simulink model "autonomous_takeoff_landing"  (Simulink 7.8)
settings: Solver=ode3  StartTime=0.0  StopTime=10.0  FixedStep=0.01  RelTol=1e-3
values from neighbouring files (symbols this model uses):
  Bkrit = 1    [parameter_ZA.m]
  Bsafe = 3    [parameter_ZA.m]
  Bstart = 5    [parameter_ZA.m]
  C_wxy = 1/2*A_xy*rho*c_w    (= 0.01986730725)    [parameter_QK.m]
  C_wz = 1/2*A_z*rho*c_w    (= 0.141396406537)    [parameter_QK.m]
  CT0 = 0.0133    [parameter_QK.m]
  CT1 = -0.0100    (= -0.01)    [parameter_QK.m]
  CT2 = 0.0081    [parameter_QK.m]
  CT3 = -0.0350    (= -0.035)    [parameter_QK.m]
  dhSinkflug = .05    (= 0.05)    [parameter_ZA.m]
  dhZulSinkflug = .05    (= 0.05)    [parameter_ZA.m]
  dSchubLanden = .05    (= 0.05)    [parameter_ZA.m]
  dSchubStart = .01    (= 0.01)    [parameter_ZA.m]
  dt = 0.01    [init.m]
  dtStart = .2    (= 0.2)    [parameter_ZA.m]
  g = 9.81    [parameter_QK.m]    (also in zulwin.m = sin(beta+pi/4)*LGB/2)
  hFlug = 1    [parameter_ZA.m]
  hLanden = LGH*4    (= 0.6)    [parameter_ZA.m]
  l_m = 0.2775    [parameter_QK.m]    (also in zulwin.m)
  LGH = 0.15    [init.m]    (also in parameter_ZA.m)
  m = 1.316    [parameter_QK.m]
  R = 0.1269    [parameter_QK.m]    (also in zulwin.m)
  rho = 1.225    [parameter_QK.m]
  SchubRun = .2    (= 0.2)    [parameter_ZA.m]
  SchubStart = 0.65    [parameter_ZA.m]
  tAnlauf = 2.5    [parameter_ZA.m]
  twc = .1    (= 0.1)    [parameter_ZA.m]
  z_m = -0.02    [parameter_QK.m]
  zpLanden = .05    (= 0.05)    [parameter_ZA.m]
  zpStart = .1    (= 0.1)    [parameter_ZA.m]
  zul_dmotor = 25    [parameter_ZA.m]
  zul_dp = .15    (= 0.15)    [parameter_ZA.m]
  zul_dwmax = 0.8    [parameter_ZA.m]
  zul_w = 2.5    [parameter_ZA.m]
  zul_win = .15    (= 0.15)    [parameter_ZA.m]
undefined symbols (not defined in the file or in its folder): Newton, Raphson
libraries: simulink x28, orocos_taskcontext x18, powerlib_extras x6, aerolibutil x4, aerolibtransform2 x1, dspmtrx3 x1
settings Model: Creator=roedelsperger  LastModifiedBy=uav
settings DebuggingCC: FcnCallInpInsideContextMsg=Use local settings
settings RTWCC: SystemTargetFile=orocos.tlc  TemplateMakefile=orocos.tmf  Description=Linux Orocos Target  ProcessScript=orocos_make_rtw_hook
settings STFCustomTargetCC: ModelReferenceCompliant=off  MatFileLogging=on  SystemTargetFile=orocos.tlc

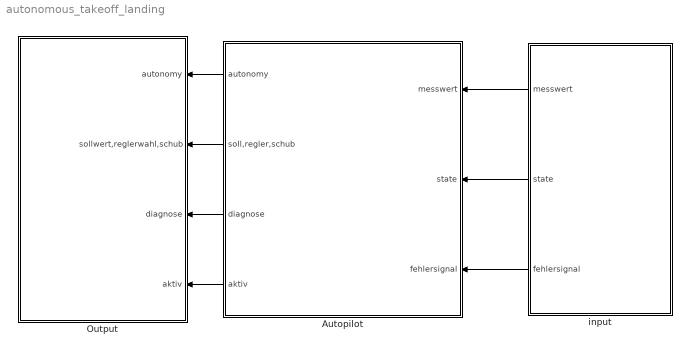
== system autonomous_takeoff_landing ==
  Autopilot : Subsystem
  Output : Subsystem
  input : Subsystem
  wires:
  input/1(messwert) -> Autopilot/1(messwert)
  input/2(state) -> Autopilot/2(state)
  Autopilot/1(autonomy) -> Output/1(autonomy)
  Autopilot/2(soll,regler,schub) -> Output/2(sollwert,reglerwahl,schub)
  Autopilot/3(diagnose) -> Output/3(diagnose)
  Autopilot/4(aktiv) -> Output/4(aktiv)
  input/3(fehlersignal) -> Autopilot/3(fehlersignal)

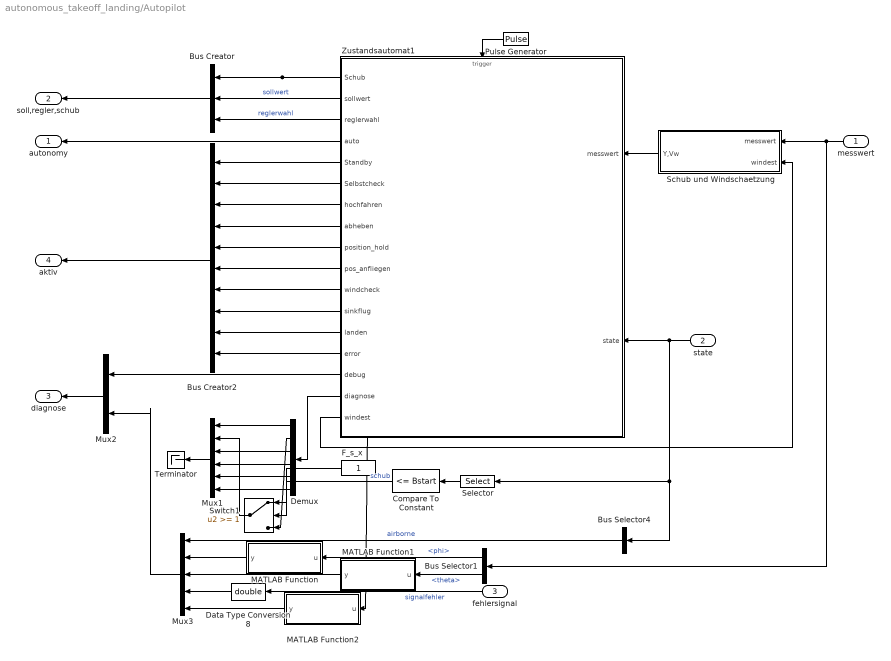
== system autonomous_takeoff_landing/Autopilot ==
  messwert : Inport
  state : Inport  Port=2
  fehlersignal : Inport  Port=3
  Bus Creator : BusCreator  Inputs=3
  Bus Creator2 : BusCreator  Inputs=10
  Bus Selector1 : BusSelector  OutputSignals=ptp.phi,ptp.theta
  Bus Selector4 : BusSelector  OutputSignals=signal5  OutputAsBus=on
  Compare To Constant : simulink/Logic and Bit Operations/Compare To Constant  relop=<=  const=Bstart  OutDataTypeStr=uint8
  Data Type Conversion8 : DataTypeConversion  OutDataTypeStr=double  RndMeth=Ceiling
  Demux : Demux  Outputs=6
  F_s_x : Constant
  MATLAB Function : MATLAB Function  TreatAsAtomicUnit=on
  MATLAB Function1 : MATLAB Function  TreatAsAtomicUnit=on
  MATLAB Function2 : MATLAB Function  TreatAsAtomicUnit=on
  Mux1 : Mux  Inputs=6
  Mux2 : Mux  Inputs=2
  Mux3 : Mux  Inputs=5
  Pulse Generator : DiscretePulseGenerator  PulseType=Time based  Period=0.02  PulseWidth=50
  Schub und Windschaetzung : Subsystem
  Selector : Selector  InputPortWidth=6  IndexOptions=Index vector (dialog)  Indices=[6]  OutputSizes=1
  Switch1 : Switch  Threshold=1
  Terminator : Terminator
  Zustandsautomat1 : Stateflow chart  TreatAsAtomicUnit=on
  autonomy : Outport
  soll,regler,schub : Outport  Port=2
  diagnose : Outport  Port=3
  aktiv : Outport  Port=4
  wires:
  messwert/1 -> Schub und Windschaetzung/1(messwert), Bus Selector1/1
  Pulse Generator/1 -> Zustandsautomat1/Trigger
  state/1 -> Zustandsautomat1/2(state), Selector/1, Bus Selector4/1
  Zustandsautomat1/1(Schub) -> Bus Creator/1, MATLAB Function2/1(u)  "schub"
  Zustandsautomat1/17(windest) -> Schub und Windschaetzung/2(windest)
  Demux/1 -> Mux1/1
  Demux/2 -> Switch1/3
  Switch1/1 -> Mux1/2
  Zustandsautomat1/16(diagnose) -> Demux/1
  Compare To Constant/1 -> Switch1/2
  Bus Creator/1 -> soll,regler,schub/1
  Zustandsautomat1/2(sollwert) -> Bus Creator/2  "sollwert"
  Zustandsautomat1/3(reglerwahl) -> Bus Creator/3  "reglerwahl"
  Zustandsautomat1/4(auto) -> autonomy/1
  Schub und Windschaetzung/1(Y,Vw) -> Zustandsautomat1/1(messwert)
  F_s_x/1 -> Switch1/1
  Selector/1 -> Compare To Constant/1
  Zustandsautomat1/5(Standby) -> Bus Creator2/1
  Zustandsautomat1/6(Selbstcheck) -> Bus Creator2/2
  Zustandsautomat1/7(hochfahren) -> Bus Creator2/3
  Zustandsautomat1/8(abheben) -> Bus Creator2/4
  Zustandsautomat1/9(position_hold) -> Bus Creator2/5
  Zustandsautomat1/10(pos_anfliegen) -> Bus Creator2/6
  Zustandsautomat1/11(windcheck) -> Bus Creator2/7
  Zustandsautomat1/12(sinkflug) -> Bus Creator2/8
  Zustandsautomat1/13(landen) -> Bus Creator2/9
  Zustandsautomat1/14(error) -> Bus Creator2/10
  Bus Creator2/1 -> aktiv/1
  Demux/3 -> Mux1/3
  Demux/4 -> Mux1/4
  Demux/5 -> Mux1/5
  Demux/6 -> Mux1/6
  Zustandsautomat1/15(debug) -> Mux2/1
  Mux2/1 -> diagnose/1
  Mux3/1 -> Mux2/2
  Mux1/1 -> Terminator/1
  fehlersignal/1 -> Data Type Conversion8/1  "signalfehler"
  Bus Selector4/1 -> Mux3/1  "airborne"
  Data Type Conversion8/1 -> Mux3/4
  MATLAB Function/1(y) -> Mux3/2
  Bus Selector1/1 -> MATLAB Function/1(u)  "<phi>"
  Bus Selector1/2 -> MATLAB Function1/1(u)  "<theta>"
  MATLAB Function1/1(y) -> Mux3/3
  MATLAB Function2/1(y) -> Mux3/5

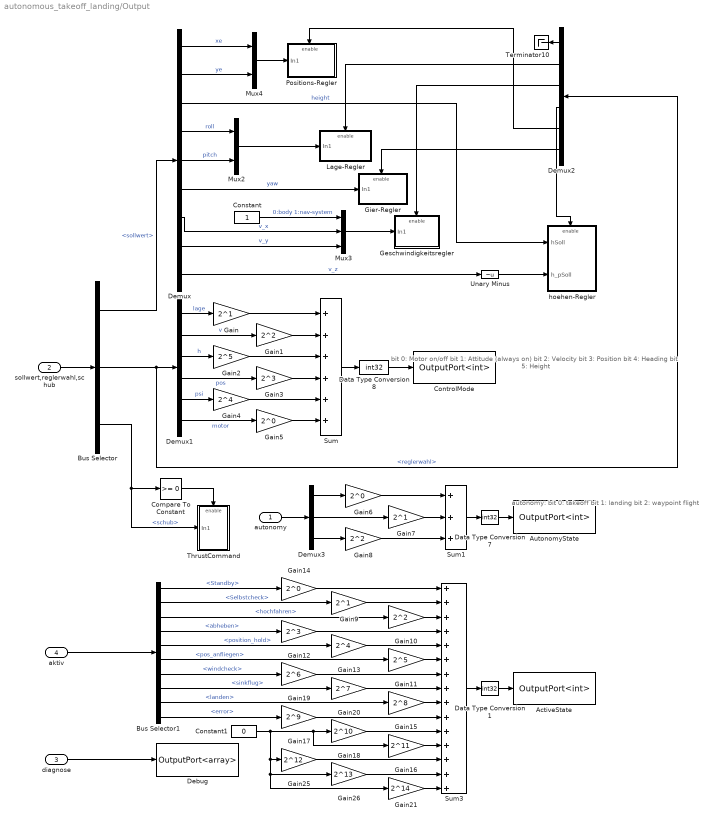
== system autonomous_takeoff_landing/Output ==
  note: bit 0: Motor on/off
      | bit 1: Attitude (always on)
      | bit 2: Velocity
      | bit 3: Position
      | bit 4: Heading
      | bit 5: Height
  note: autonomy:
      |   bit 0: takeoff
      |   bit 1: landing
      |   bit 2: waypoint flight
  autonomy : Inport
  sollwert,reglerwahl,schub : Inport  Port=2
  diagnose : Inport  Port=3
  aktiv : Inport  Port=4
  ActiveState : orocos_taskcontext/OutputPort<int>  dpdesc=Port's Description  dpvalue=0
      settings: AttributesFormatString=Value=%<dpvalue>
  AutonomyState : orocos_taskcontext/OutputPort<int>  dpdesc=Port's Description  dpvalue=0
      settings: AttributesFormatString=Value=%<dpvalue>
  Bus Selector : BusSelector  OutputSignals=sollwert,reglerwahl,schub
  Bus Selector1 : BusSelector  OutputSignals=Standby,Selbstcheck,hochfahren,abheben,position_hold,pos_anfliegen,windcheck,sinkflug,landen,error
  Compare To Constant : simulink/Logic and Bit Operations/Compare To Constant  relop=>=  const=0  OutDataTypeStr=uint8
  Constant : Constant
  Constant1 : Constant  Value=0
  ControlMode : orocos_taskcontext/OutputPort<int>  dpdesc=Port's Description  dpvalue=0
      settings: AttributesFormatString=Value=%<dpvalue>
  Data Type Conversion1 : DataTypeConversion  OutDataTypeStr=int32  RndMeth=Ceiling
  Data Type Conversion7 : DataTypeConversion  OutDataTypeStr=int32  RndMeth=Ceiling
  Data Type Conversion8 : DataTypeConversion  OutDataTypeStr=int32  RndMeth=Ceiling
  Debug : orocos_taskcontext/OutputPort<array>  dpdesc=Port's Description  dpvalue=[0.0]
      settings: AttributesFormatString=Value=%<dpvalue>
  Demux : Demux  Outputs=9
  Demux1 : Demux  Outputs=6
  Demux2 : Demux  Outputs=6
  Demux3 : Demux  Outputs=3
  Gain : Gain  Gain=2^1
  Gain1 : Gain  Gain=2^2
  Gain10 : Gain  Gain=2^2
  Gain11 : Gain  Gain=2^5
  Gain12 : Gain  Gain=2^3
  Gain13 : Gain  Gain=2^4
  Gain14 : Gain  Gain=2^0
  Gain15 : Gain  Gain=2^8
  Gain16 : Gain  Gain=2^11
  Gain17 : Gain  Gain=2^9
  Gain18 : Gain  Gain=2^10
  Gain19 : Gain  Gain=2^6
  Gain2 : Gain  Gain=2^5
  Gain20 : Gain  Gain=2^7
  Gain21 : Gain  Gain=2^14
  Gain25 : Gain  Gain=2^12
  Gain26 : Gain  Gain=2^13
  Gain3 : Gain  Gain=2^3
  Gain4 : Gain  Gain=2^4
  Gain5 : Gain  Gain=2^0
  Gain6 : Gain  Gain=2^0
  Gain7 : Gain  Gain=2^1
  Gain8 : Gain  Gain=2^2
  Gain9 : Gain  Gain=2^1
  Geschwindigkeitsregler : Subsystem
  Gier-Regler : Subsystem
  Lage-Regler : Subsystem
  Mux2 : Mux  Inputs=2
  Mux3 : Mux  Inputs=3
  Mux4 : Mux  Inputs=2
  Positions-Regler : Subsystem
  Sum : Sum  Inputs=++++++
  Sum1 : Sum  Inputs=+++
  Sum3 : Sum  Inputs=+++++++++++++++
  Terminator10 : Terminator
  ThrustCommand : Subsystem
  Unary Minus : UnaryMinus
  hoehen-Regler : Subsystem
  wires:
  sollwert,reglerwahl,schub/1 -> Bus Selector/1
  Bus Selector/1 -> Demux/1  "<sollwert>"
  Mux2/1 -> Lage-Regler/1(In1)
  Demux/4 -> Mux2/1  "roll"
  Demux/5 -> Mux2/2  "pitch"
  Demux/6 -> Gier-Regler/1(In1)  "yaw"
  Mux3/1 -> Geschwindigkeitsregler/1(In1)
  Constant/1 -> Mux3/1  "0:body 1:nav-system"
  Demux/7 -> Mux3/2  "v_x"
  Demux/8 -> Mux3/3  "v_y"
  Demux/3 -> hoehen-Regler/1(hSoll)  "height"
  Demux/9 -> Unary Minus/1  "v_z"
  Demux/1 -> Mux4/1  "xe"
  Demux/2 -> Mux4/2  "ye"
  Mux4/1 -> Positions-Regler/1(In1)
  Demux2/1 -> Terminator10/1
  Demux2/2 -> Lage-Regler/Enable
  Demux2/3 -> Geschwindigkeitsregler/Enable
  Demux2/4 -> hoehen-Regler/Enable
  Demux2/5 -> Positions-Regler/Enable
  Demux2/6 -> Gier-Regler/Enable
  Compare To Constant/1 -> ThrustCommand/Enable
  Bus Selector/2 -> Demux1/1, Demux2/1  "<reglerwahl>"
  Unary Minus/1 -> hoehen-Regler/2(h_pSoll)
  Demux1/1 -> Gain/1  "lage"
  Demux1/2 -> Gain1/1  "v"
  Demux1/3 -> Gain2/1  "h"
  Demux1/4 -> Gain3/1  "pos"
  Demux1/5 -> Gain4/1  "psi"
  Demux1/6 -> Gain5/1  "motor"
  Gain6/1 -> Sum1/1
  Gain7/1 -> Sum1/2
  Gain8/1 -> Sum1/3
  Sum1/1 -> Data Type Conversion7/1
  Demux3/1 -> Gain6/1
  Demux3/2 -> Gain7/1
  Demux3/3 -> Gain8/1
  autonomy/1 -> Demux3/1
  Bus Selector/3 -> Compare To Constant/1, ThrustCommand/1(In1)  "<schub>"
  Sum/1 -> Data Type Conversion8/1
  Data Type Conversion7/1 -> AutonomyState/1
  Data Type Conversion8/1 -> ControlMode/1
  Gain/1 -> Sum/1
  Gain1/1 -> Sum/2
  Gain2/1 -> Sum/3
  Gain3/1 -> Sum/4
  Gain4/1 -> Sum/5
  Gain5/1 -> Sum/6
  aktiv/1 -> Bus Selector1/1
  Sum3/1 -> Data Type Conversion1/1
  Data Type Conversion1/1 -> ActiveState/1
  Bus Selector1/1 -> Gain14/1  "<Standby>"
  Bus Selector1/2 -> Gain9/1  "<Selbstcheck>"
  Bus Selector1/3 -> Gain10/1  "<hochfahren>"
  Bus Selector1/4 -> Gain12/1  "<abheben>"
  Bus Selector1/5 -> Gain13/1  "<position_hold>"
  Bus Selector1/6 -> Gain11/1  "<pos_anfliegen>"
  Bus Selector1/7 -> Gain19/1  "<windcheck>"
  Bus Selector1/8 -> Gain20/1  "<sinkflug>"
  Bus Selector1/9 -> Gain15/1  "<landen>"
  Bus Selector1/10 -> Gain17/1  "<error>"
  Gain14/1 -> Sum3/1
  Gain9/1 -> Sum3/2
  Gain10/1 -> Sum3/3
  Gain12/1 -> Sum3/4
  Gain13/1 -> Sum3/5
  Gain11/1 -> Sum3/6
  Gain19/1 -> Sum3/7
  Gain20/1 -> Sum3/8
  Gain15/1 -> Sum3/9
  Gain17/1 -> Sum3/10
  Gain18/1 -> Sum3/11
  Gain16/1 -> Sum3/12
  Gain25/1 -> Sum3/13
  Gain26/1 -> Sum3/14
  Gain21/1 -> Sum3/15
  diagnose/1 -> Debug/1
  Constant1/1 -> Gain18/1, Gain16/1, Gain25/1, Gain26/1, Gain21/1

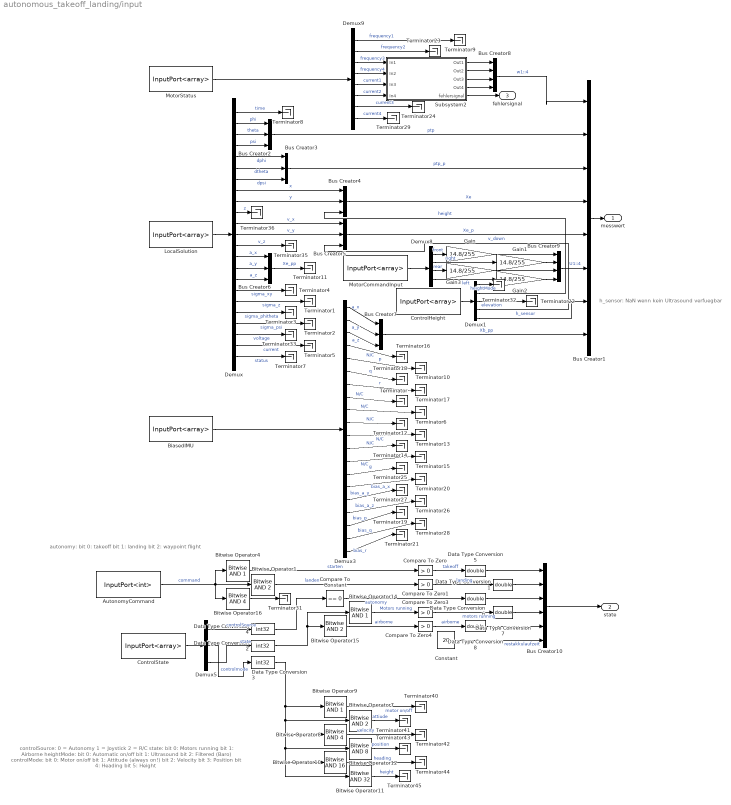
== system autonomous_takeoff_landing/input ==
  note: autonomy:
      |   bit 0: takeoff
      |   bit 1: landing
      |   bit 2: waypoint flight
  note: controlSource:
      |   0 = Autonomy
      |   1 = Joystick
      |   2 = R/C
      | state:
      |   bit 0: Motors running
      |   bit 1: Airborne
      | heightMode:
      |   bit 0: Automatic on/off
      |   bit 1: Ultrasound
      |   bit 2: Filtered (Baro)
      | controlMode:
      |   bit 0: Motor on/off
      |   bit 1: Attitude (always on!)
      |   bit 2: Velocity
      |   bit 3: Position
      |   bit 4: Heading
      |   bit 5: Height
  note: h_sensor: NaN wenn kein Ultrasound verfuegbar
  AutonomyCommand : orocos_taskcontext/InputPort<int>  dpdesc=Port's Description  dpvalue=0
      settings: AttributesFormatString=Value=%<dpvalue>
  BiasedIMU : orocos_taskcontext/InputPort<array>  dpdesc=Port's Description  dpvalue=zeros(1,20)
      settings: AttributesFormatString=Value=%<dpvalue>
  Bitwise Operator1 : simulink/Logic and Bit Operations/Bitwise Operator  logicop=AND  UseBitMask=on  BitMask=2  BitMaskRealWorld=Stored Integer
  Bitwise Operator10 : simulink/Logic and Bit Operations/Bitwise Operator  logicop=AND  UseBitMask=on  BitMask=16  BitMaskRealWorld=Stored Integer
  Bitwise Operator11 : simulink/Logic and Bit Operations/Bitwise Operator  logicop=AND  UseBitMask=on  BitMask=32  BitMaskRealWorld=Stored Integer
  Bitwise Operator12 : simulink/Logic and Bit Operations/Bitwise Operator  logicop=AND  UseBitMask=on  BitMask=8  BitMaskRealWorld=Stored Integer
  Bitwise Operator14 : simulink/Logic and Bit Operations/Bitwise Operator  logicop=AND  UseBitMask=on  BitMask=1  BitMaskRealWorld=Stored Integer
  Bitwise Operator15 : simulink/Logic and Bit Operations/Bitwise Operator  logicop=AND  UseBitMask=on  BitMask=2  BitMaskRealWorld=Stored Integer
  Bitwise Operator16 : simulink/Logic and Bit Operations/Bitwise Operator  logicop=AND  UseBitMask=on  BitMask=4  BitMaskRealWorld=Stored Integer
  Bitwise Operator4 : simulink/Logic and Bit Operations/Bitwise Operator  logicop=AND  UseBitMask=on  BitMask=1  BitMaskRealWorld=Stored Integer
  Bitwise Operator7 : simulink/Logic and Bit Operations/Bitwise Operator  logicop=AND  UseBitMask=on  BitMask=2  BitMaskRealWorld=Stored Integer
  Bitwise Operator8 : simulink/Logic and Bit Operations/Bitwise Operator  logicop=AND  UseBitMask=on  BitMask=4  BitMaskRealWorld=Stored Integer
  Bitwise Operator9 : simulink/Logic and Bit Operations/Bitwise Operator  logicop=AND  UseBitMask=on  BitMask=1  BitMaskRealWorld=Stored Integer
  Bus Creator1 : BusCreator  Inputs=8
  Bus Creator10 : BusCreator  Inputs=6
  Bus Creator{2..7} (6 alike) : BusCreator  Inputs=3
  Bus Creator8 : BusCreator
  Bus Creator9 : BusCreator
  Compare To Constant : simulink/Logic and Bit Operations/Compare To Constant  relop===  const=0  OutDataTypeStr=boolean
  Compare To Zero{,1,3..4} (4 alike) : simulink/Logic and Bit Operations/Compare To Zero  relop=>  OutDataTypeStr=boolean
  Constant : Constant  Value=20
  ControlHeight : orocos_taskcontext/InputPort<array>  dpdesc=Port's Description  dpvalue=zeros(1,5)
      settings: AttributesFormatString=Value=%<dpvalue>
  ControlState : orocos_taskcontext/InputPort<array>  dpdesc=Port's Description  dpvalue=zeros(1,3)
      settings: AttributesFormatString=Value=%<dpvalue>
  Data Type Conversion{1,5..8} (5 alike) : DataTypeConversion  OutDataTypeStr=double  RndMeth=Ceiling
  Data Type Conversion2 : DataTypeConversion  OutDataTypeStr=int32  RndMeth=Ceiling
  Data Type Conversion3 : DataTypeConversion  OutDataTypeStr=int32  RndMeth=Ceiling
  Data Type Conversion4 : DataTypeConversion  OutDataTypeStr=int32  RndMeth=Ceiling
  Demux : Demux  Outputs=23
  Demux1 : Demux  Outputs=5
  Demux3 : Demux  Outputs=20
  Demux5 : Demux  Outputs=3
  Demux8 : Demux
  Demux9 : Demux  Outputs=8
  Gain{,1..3} (4 alike) : Gain  Gain=14.8/255
  LocalSolution : orocos_taskcontext/InputPort<array>  dpdesc=Port's Description  dpvalue=zeros(1,23)
      settings: AttributesFormatString=Value=%<dpvalue>
  MotorCommandInput : orocos_taskcontext/InputPort<array>  dpdesc=Port's Description  dpvalue=zeros(1,4)
      settings: AttributesFormatString=Value=%<dpvalue>
  MotorStatus : orocos_taskcontext/InputPort<array>  dpdesc=Port's Description  dpvalue=zeros(1,8)
      settings: AttributesFormatString=Value=%<dpvalue>
  Subsystem2 : Subsystem
  Terminator{,1..29,31..33,35..36,40..45} (41 alike) : Terminator
  messwert : Outport
  state : Outport  Port=2
  fehlersignal : Outport  Port=3
  wires:
  LocalSolution/1 -> Demux/1
  ControlState/1 -> Demux5/1
  Demux/1 -> Terminator8/1  "time"
  Demux/2 -> Bus Creator2/1  "phi"
  Demux/3 -> Bus Creator2/2  "theta"
  Demux/4 -> Bus Creator2/3  "psi"
  Demux/5 -> Bus Creator3/1  "dphi"
  Demux/6 -> Bus Creator3/2  "dtheta"
  Demux/7 -> Bus Creator3/3  "dpsi"
  Demux/8 -> Bus Creator4/1  "x"
  Demux/9 -> Bus Creator4/2  "y"
  Demux/11 -> Bus Creator5/1  "v_x"
  Demux/12 -> Bus Creator5/2  "v_y"
  Demux/14 -> Bus Creator6/1  "a_x"
  Demux/15 -> Bus Creator6/2  "a_y"
  Demux/16 -> Bus Creator6/3  "a_z"
  Demux/17 -> Terminator4/1  "sigma_xy"
  Demux/18 -> Terminator1/1  "sigma_z"
  Demux/19 -> Terminator3/1  "sigma_phitheta"
  Demux/20 -> Terminator2/1  "sigma_psi"
  Demux/21 -> Terminator33/1  "voltage"
  Demux/22 -> Terminator5/1  "current"
  Demux/23 -> Terminator7/1  "status"
  Demux5/1 -> Data Type Conversion4/1  "controlSource"
  Bus Creator1/1 -> messwert/1
  Bus Creator2/1 -> Bus Creator1/2  "ptp"
  Bus Creator6/1 -> Terminator11/1  "Xe_pp"
  BiasedIMU/1 -> Demux3/1
  Demux3/1 -> Bus Creator7/1  "a_x"
  Demux3/2 -> Bus Creator7/2  "a_y"
  Demux3/3 -> Bus Creator7/3  "a_z"
  Demux3/4 -> Terminator16/1  "N/C"
  Demux3/5 -> Terminator10/1  "p"
  Demux3/6 -> Terminator18/1  "q"
  Demux3/7 -> Terminator17/1  "r"
  Demux3/8 -> Terminator/1  "N/C"
  Demux3/9 -> Terminator6/1  "N/C"
  Demux3/10 -> Terminator12/1  "N/C"
  Demux3/11 -> Terminator13/1  "N/C"
  Demux3/12 -> Terminator14/1  "N/C"
  Demux3/13 -> Terminator15/1  "N/C"
  Demux3/14 -> Terminator25/1  "g"
  Demux3/15 -> Terminator20/1  "bias_a_x"
  Demux3/16 -> Terminator27/1  "bias_a_y"
  Demux3/17 -> Terminator26/1  "bias_a_z"
  Demux3/18 -> Terminator19/1  "bias_p"
  Demux3/19 -> Terminator28/1  "bias_q"
  Demux3/20 -> Terminator21/1  "bias_r"
  Bus Creator5/1 -> Bus Creator1/5  "Xe_p"
  Bus Creator4/1 -> Bus Creator1/4  "Xe"
  Bus Creator3/1 -> Bus Creator1/3  "ptp_p"
  MotorStatus/1 -> Demux9/1
  Bus Creator8/1 -> Bus Creator1/1  "w1::4"
  MotorCommandInput/1 -> Demux8/1
  Bus Creator9/1 -> Bus Creator1/6  "U1::4"
  Bus Creator7/1 -> Bus Creator1/8  "Xb_pp"
  AutonomyCommand/1 -> Bitwise Operator4/1, Bitwise Operator1/1, Bitwise Operator16/1  "command"
  Bitwise Operator16/1 -> Terminator31/1
  Bitwise Operator1/1 -> Compare To Zero1/1  "landen"
  Bitwise Operator4/1 -> Compare To Zero/1  "starten"
  Bitwise Operator9/1 -> Terminator40/1  "motor on/off"
  Bitwise Operator7/1 -> Terminator41/1  "attiude"
  Bitwise Operator8/1 -> Terminator42/1  "velocity"
  Bitwise Operator12/1 -> Terminator43/1  "position"
  Bitwise Operator10/1 -> Terminator44/1  "heading"
  Bitwise Operator11/1 -> Terminator45/1  "height"
  Demux1/1 -> Terminator32/1  "heightMode"
  Demux1/3 -> Terminator22/1  "elevation"
  ControlHeight/1 -> Demux1/1
  Bitwise Operator14/1 -> Compare To Zero3/1  "Motors running"
  Bitwise Operator15/1 -> Compare To Zero4/1  "airborne"
  Demux/13 -> Terminator35/1  "v_z"
  Demux/10 -> Terminator36/1  "z"
  Bus Creator10/1 -> state/1
  Demux1/4 -> Bus Creator5/3  "v_down"
  Demux1/2 -> Bus Creator4/3  "height"
  Demux1/5 -> Bus Creator1/7  "h_sensor"
  Data Type Conversion2/1 -> Bitwise Operator14/1, Bitwise Operator15/1
  Data Type Conversion3/1 -> Bitwise Operator9/1, Bitwise Operator8/1, Bitwise Operator12/1, Bitwise Operator10/1, Bitwise Operator11/1, Bitwise Operator7/1
  Compare To Zero/1 -> Data Type Conversion5/1  "takeoff"
  Compare To Zero1/1 -> Data Type Conversion1/1  "landing"
  Compare To Zero3/1 -> Data Type Conversion7/1  "motors running"
  Compare To Zero4/1 -> Data Type Conversion8/1  "airborne"
  Data Type Conversion4/1 -> Compare To Constant/1
  Compare To Constant/1 -> Data Type Conversion6/1  "autonomy"
  Constant/1 -> Bus Creator10/6  "restakkulaufzeit"
  Data Type Conversion5/1 -> Bus Creator10/1
  Data Type Conversion1/1 -> Bus Creator10/2
  Data Type Conversion6/1 -> Bus Creator10/3
  Data Type Conversion7/1 -> Bus Creator10/4
  Data Type Conversion8/1 -> Bus Creator10/5
  Demux8/1 -> Gain/1  "front"
  Demux8/2 -> Gain1/1  "right"
  Demux8/3 -> Gain3/1  "rear"
  Demux8/4 -> Gain2/1  "left"
  Gain/1 -> Bus Creator9/1
  Gain1/1 -> Bus Creator9/2
  Gain3/1 -> Bus Creator9/3
  Gain2/1 -> Bus Creator9/4
  Demux5/3 -> Data Type Conversion2/1  "state"
  Demux5/2 -> Data Type Conversion3/1  "controlmode"
  Demux9/1 -> Terminator9/1  "frequency1"
  Demux9/2 -> Terminator23/1  "frequency2"
  Demux9/7 -> Terminator24/1  "current3"
  Demux9/8 -> Terminator29/1  "current4"
  Demux9/3 -> Subsystem2/1(In1)  "frequency3"
  Demux9/4 -> Subsystem2/2(In2)  "frequency4"
  Demux9/5 -> Subsystem2/3(In3)  "current1"
  Demux9/6 -> Subsystem2/4(In4)  "current2"
  Subsystem2/1(Out1) -> Bus Creator8/1
  Subsystem2/2(Out2) -> Bus Creator8/2
  Subsystem2/3(Out3) -> Bus Creator8/3
  Subsystem2/4(Out4) -> Bus Creator8/4
  Subsystem2/5(fehlersignal) -> fehlersignal/1

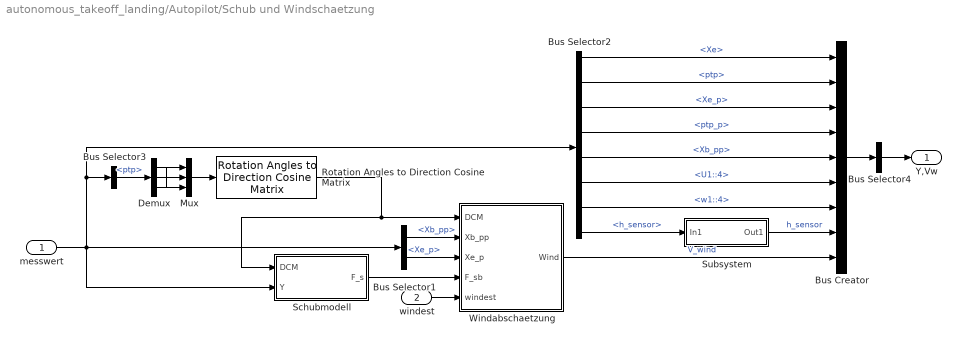
== system autonomous_takeoff_landing/Autopilot/Schub und Windschaetzung ==
  messwert : Inport
  windest : Inport  Port=2
  Bus Creator : BusCreator  Inputs=9
  Bus Selector1 : BusSelector  OutputSignals=Xb_pp,Xe_p
  Bus Selector2 : BusSelector  OutputSignals=Xe,ptp,Xe_p,ptp_p,Xb_pp,U1::4,w1::4,h_sensor
  Bus Selector3 : BusSelector  OutputSignals=ptp
  Bus Selector4 : BusSelector  OutputSignals=Xe,ptp,Xe_p,ptp_p,h_sensor,w1::4,V_wind  OutputAsBus=on
  Demux : Demux  Outputs=3
  Mux : Mux  Inputs=3
  Rotation Angles to Direction Cosine Matrix : aerolibtransform2/Rotation Angles to Direction Cosine Matrix  rotationOrder=ZYX
  Schubmodell : Subsystem
  Subsystem : Subsystem
  Windabschaetzung : Subsystem
  Y,Vw : Outport
  wires:
  Schubmodell/1(F_s) -> Windabschaetzung/4(F_sb)
  Bus Selector1/1 -> Windabschaetzung/2(Xb_pp)  "<Xb_pp>"
  Bus Selector1/2 -> Windabschaetzung/3(Xe_p)  "<Xe_p>"
  messwert/1 -> Bus Selector1/1, Bus Selector2/1, Bus Selector3/1, Schubmodell/2(Y)
  Bus Selector2/1 -> Bus Creator/1  "<Xe>"
  Bus Selector2/2 -> Bus Creator/2  "<ptp>"
  Bus Selector2/3 -> Bus Creator/3  "<Xe_p>"
  Bus Selector2/4 -> Bus Creator/4  "<ptp_p>"
  Windabschaetzung/1(Wind) -> Bus Creator/9  "V_wind"
  windest/1 -> Windabschaetzung/5(windest)
  Bus Selector2/5 -> Bus Creator/5  "<Xb_pp>"
  Bus Selector2/6 -> Bus Creator/6  "<U1::4>"
  Bus Selector2/7 -> Bus Creator/7  "<w1::4>"
  Bus Selector2/8 -> Subsystem/1(In1)  "<h_sensor>"
  Mux/1 -> Rotation Angles to Direction Cosine Matrix/1
  Bus Selector3/1 -> Demux/1  "<ptp>"
  Demux/2 -> Mux/2
  Demux/1 -> Mux/3
  Demux/3 -> Mux/1
  Rotation Angles to Direction Cosine Matrix/1 -> Windabschaetzung/1(DCM), Schubmodell/1(DCM)
  Bus Creator/1 -> Bus Selector4/1
  Bus Selector4/1 -> Y,Vw/1
  Subsystem/1(Out1) -> Bus Creator/8  "h_sensor"

== system autonomous_takeoff_landing/Output/Geschwindigkeitsregler ==
  In1 : Inport
  Enable : EnablePort
  VelocityCommandOutput : orocos_taskcontext/OutputPort<array>  dpdesc=Port's Description  dpvalue=zeros(1,2)
      settings: AttributesFormatString=Value=%<dpvalue>
  wires:
  In1/1 -> VelocityCommandOutput/1

== system autonomous_takeoff_landing/Output/Gier-Regler ==
  In1 : Inport
  Enable : EnablePort
  HeadingCommandOutput : orocos_taskcontext/OutputPort<array>  dpdesc=Port's Description  dpvalue=0.0
      settings: AttributesFormatString=Value=%<dpvalue>
  wires:
  In1/1 -> HeadingCommandOutput/1

== system autonomous_takeoff_landing/Output/Lage-Regler ==
  In1 : Inport
  Enable : EnablePort
  AttitudeCommandOutput : orocos_taskcontext/OutputPort<array>  dpdesc=Port's Description  dpvalue=zeros(1,2)
      settings: AttributesFormatString=Value=%<dpvalue>
  wires:
  In1/1 -> AttitudeCommandOutput/1

== system autonomous_takeoff_landing/Output/Positions-Regler ==
  In1 : Inport
  Enable : EnablePort
  PositionCommandOutput : orocos_taskcontext/OutputPort<array>  dpdesc=Port's Description  dpvalue=zeros(1,2)
      settings: AttributesFormatString=Value=%<dpvalue>
  wires:
  In1/1 -> PositionCommandOutput/1

== system autonomous_takeoff_landing/Output/ThrustCommand ==
  In1 : Inport
  Enable : EnablePort
  ThrustCommandOutput : orocos_taskcontext/OutputPort<array>  dpdesc=Port's Description  dpvalue=0.0
      settings: AttributesFormatString=Value=%<dpvalue>
  wires:
  In1/1 -> ThrustCommandOutput/1

== system autonomous_takeoff_landing/Output/hoehen-Regler ==
  hSoll : Inport
  h_pSoll : Inport  Port=2
  Enable : EnablePort
  ClimbrateCommandOutput : orocos_taskcontext/OutputPort<array>  dpdesc=Port's Description  dpvalue=0.0
      settings: AttributesFormatString=Value=%<dpvalue>
  HeightCommandOutput : orocos_taskcontext/OutputPort<array>  dpdesc=Port's Description  dpvalue=0.0
      settings: AttributesFormatString=Value=%<dpvalue>
  wires:
  hSoll/1 -> HeightCommandOutput/1
  h_pSoll/1 -> ClimbrateCommandOutput/1

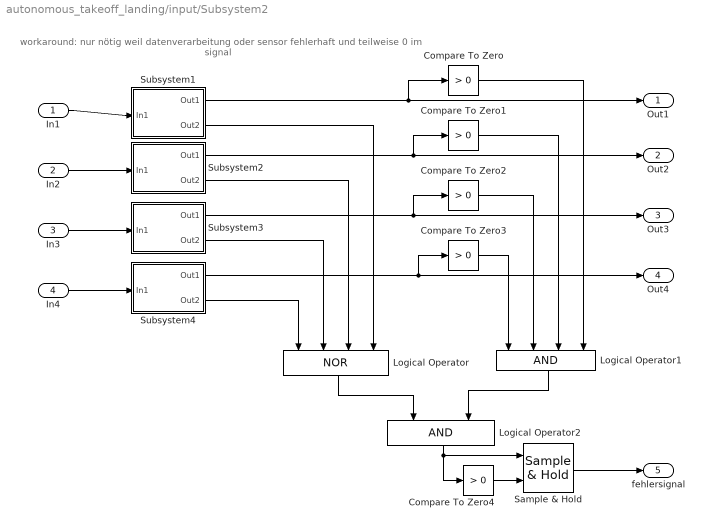
== system autonomous_takeoff_landing/input/Subsystem2 ==
  note: workaround: nur nötig weil datenverarbeitung oder sensor fehlerhaft
      | und teilweise 0 im signal
  In1 : Inport
  In2 : Inport  Port=2
  In3 : Inport  Port=3
  In4 : Inport  Port=4
  Compare To Zero{,1..4} (5 alike) : simulink/Logic and Bit Operations/Compare To Zero  relop=>  OutDataTypeStr=uint8
  Logical Operator : Logic  Operator=NOR  Inputs=4  AllPortsSameDT=off  OutDataTypeStr=boolean
  Logical Operator1 : Logic  Inputs=4  AllPortsSameDT=off  OutDataTypeStr=boolean
  Logical Operator2 : Logic  AllPortsSameDT=off  OutDataTypeStr=boolean
  Sample & Hold : powerlib_extras/Control  Blocks/Sample & Hold  ic=0
  Subsystem1 : Subsystem
  Subsystem2 : Subsystem
  Subsystem3 : Subsystem
  Subsystem4 : Subsystem
  Out1 : Outport
  Out2 : Outport  Port=2
  Out3 : Outport  Port=3
  Out4 : Outport  Port=4
  fehlersignal : Outport  Port=5
  wires:
  Subsystem1/1(Out1) -> Out1/1, Compare To Zero/1
  In1/1 -> Subsystem1/1(In1)
  In2/1 -> Subsystem2/1(In1)
  Subsystem2/1(Out1) -> Out2/1, Compare To Zero1/1
  In3/1 -> Subsystem3/1(In1)
  Subsystem3/1(Out1) -> Out3/1, Compare To Zero2/1
  In4/1 -> Subsystem4/1(In1)
  Subsystem4/1(Out1) -> Out4/1, Compare To Zero3/1
  Compare To Zero/1 -> Logical Operator1/4
  Compare To Zero1/1 -> Logical Operator1/3
  Compare To Zero2/1 -> Logical Operator1/2
  Compare To Zero3/1 -> Logical Operator1/1
  Subsystem1/2(Out2) -> Logical Operator/4
  Subsystem2/2(Out2) -> Logical Operator/3
  Subsystem3/2(Out2) -> Logical Operator/2
  Subsystem4/2(Out2) -> Logical Operator/1
  Logical Operator/1 -> Logical Operator2/1
  Logical Operator1/1 -> Logical Operator2/2
  Logical Operator2/1 -> Sample & Hold/1, Compare To Zero4/1
  Sample & Hold/1 -> fehlersignal/1
  Compare To Zero4/1 -> Sample & Hold/2

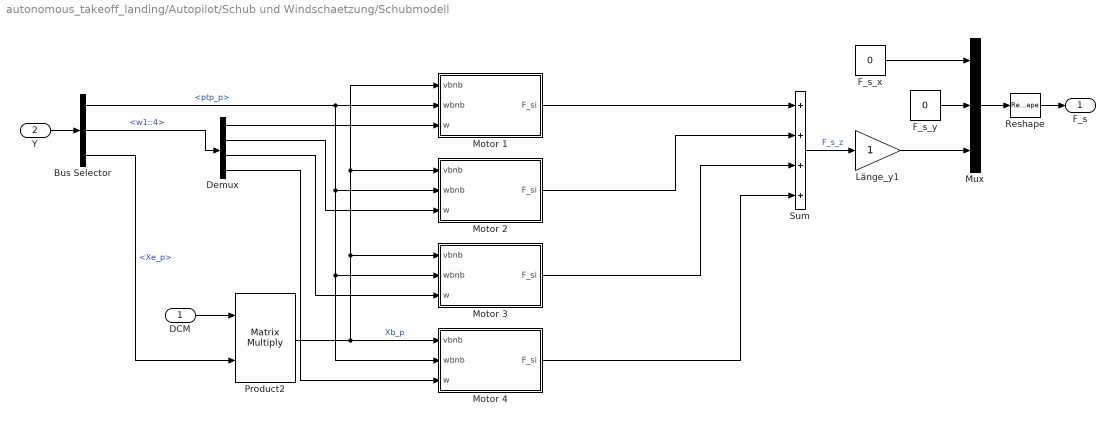
== system autonomous_takeoff_landing/Autopilot/Schub und Windschaetzung/Schubmodell ==
  DCM : Inport
  Y : Inport  Port=2
  Bus Selector : BusSelector  OutputSignals=ptp_p,w1::4,Xe_p
  Demux : Demux
  F_s_x : Constant  Value=0
  F_s_y : Constant  Value=0
  Länge_y1 : Gain
  Motor 1 : Subsystem
  Motor 2 : Subsystem
  Motor 3 : Subsystem
  Motor 4 : Subsystem
  Mux : Mux  Inputs=3
  Product2 : Product  Multiplication=Matrix(*)  RndMeth=Zero
  Reshape : Reshape
  Sum : Sum  Inputs=++++
  F_s : Outport
  wires:
  Sum/1 -> Länge_y1/1  "F_s_z"
  F_s_y/1 -> Mux/2
  F_s_x/1 -> Mux/1
  Mux/1 -> Reshape/1
  Reshape/1 -> F_s/1
  Länge_y1/1 -> Mux/3
  Bus Selector/1 -> Motor 1/2(wbnb), Motor 3/2(wbnb), Motor 4/2(wbnb), Motor 2/2(wbnb)  "<ptp_p>"
  Motor 1/1(F_si) -> Sum/1
  Bus Selector/3 -> Product2/2  "<Xe_p>"
  DCM/1 -> Product2/1
  Product2/1 -> Motor 1/1(vbnb), Motor 2/1(vbnb), Motor 3/1(vbnb), Motor 4/1(vbnb)  "Xb_p"
  Y/1 -> Bus Selector/1
  Bus Selector/2 -> Demux/1  "<w1::4>"
  Demux/1 -> Motor 1/3(w)
  Demux/2 -> Motor 2/3(w)
  Demux/3 -> Motor 3/3(w)
  Demux/4 -> Motor 4/3(w)
  Motor 2/1(F_si) -> Sum/2
  Motor 3/1(F_si) -> Sum/3
  Motor 4/1(F_si) -> Sum/4

== system autonomous_takeoff_landing/Autopilot/Schub und Windschaetzung/Subsystem ==
  In1 : Inport
  Constant : Constant  Value=10
  Logical Operator : Logic  Operator=OR  AllPortsSameDT=off  OutDataTypeStr=boolean
  Relational Operator : RelationalOperator  Operator=isInf  OutDataTypeStr=boolean
  Relational Operator1 : RelationalOperator  Operator=isNaN  OutDataTypeStr=boolean
  Switch : Switch  Criteria=u2 > Threshold
  Out1 : Outport
  wires:
  In1/1 -> Relational Operator/1, Relational Operator1/1, Switch/3
  Relational Operator/1 -> Logical Operator/1
  Relational Operator1/1 -> Logical Operator/2
  Logical Operator/1 -> Switch/2
  Switch/1 -> Out1/1
  Constant/1 -> Switch/1

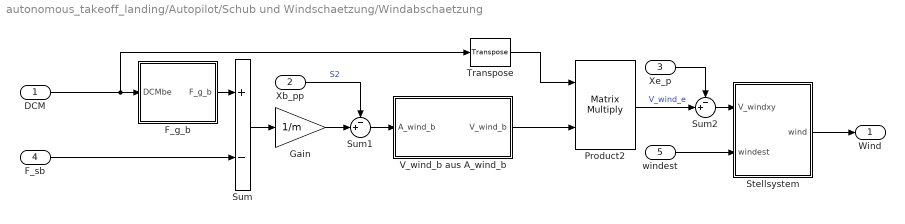
== system autonomous_takeoff_landing/Autopilot/Schub und Windschaetzung/Windabschaetzung ==
  DCM : Inport
  Xb_pp : Inport  Port=2
  Xe_p : Inport  Port=3
  F_sb : Inport  Port=4
  windest : Inport  Port=5
  F_g_b : Subsystem
  Gain : Gain  Gain=1/m
  Product2 : Product  Multiplication=Matrix(*)  RndMeth=Zero
  Stellsystem : Subsystem
  Sum : Sum  Inputs=+-
  Sum1 : Sum  Inputs=-+|
  Sum2 : Sum  Inputs=-+|
  Transpose : dspmtrx3/Transpose  Hermitian=off  overflowFlag=off
  V_wind_b aus A_wind_b : Subsystem
  Wind : Outport
  wires:
  Sum/1 -> Gain/1
  Sum1/1 -> V_wind_b aus A_wind_b/1(A_wind_b)
  Gain/1 -> Sum1/2
  F_g_b/1(F_g_b) -> Sum/1
  Stellsystem/1(wind) -> Wind/1
  Sum2/1 -> Stellsystem/1(V_windxy)
  F_sb/1 -> Sum/2
  Xb_pp/1 -> Sum1/1  "S2"
  windest/1 -> Stellsystem/2(windest)
  DCM/1 -> F_g_b/1(DCMbe), Transpose/1
  V_wind_b aus A_wind_b/1(V_wind_b) -> Product2/2
  Transpose/1 -> Product2/1
  Xe_p/1 -> Sum2/1
  Product2/1 -> Sum2/2  "V_wind_e"

== system autonomous_takeoff_landing/input/Subsystem2/Subsystem1 ==
  In1 : Inport
  Compare To Constant1 : simulink/Logic and Bit Operations/Compare To Constant  relop=~=  const=0  OutDataTypeStr=uint8
  Sample & Hold : powerlib_extras/Control  Blocks/Sample & Hold  ic=0
  Out1 : Outport
  Out2 : Outport  Port=2
  wires:
  Sample & Hold/1 -> Out1/1
  In1/1 -> Sample & Hold/1, Compare To Constant1/1
  Compare To Constant1/1 -> Sample & Hold/2, Out2/1

== system autonomous_takeoff_landing/input/Subsystem2/Subsystem2 ==
  In1 : Inport
  Compare To Constant1 : simulink/Logic and Bit Operations/Compare To Constant  relop=~=  const=0  OutDataTypeStr=uint8
  Sample & Hold : powerlib_extras/Control  Blocks/Sample & Hold  ic=0
  Out1 : Outport
  Out2 : Outport  Port=2
  wires:
  Sample & Hold/1 -> Out1/1
  In1/1 -> Sample & Hold/1, Compare To Constant1/1
  Compare To Constant1/1 -> Sample & Hold/2, Out2/1

== system autonomous_takeoff_landing/input/Subsystem2/Subsystem3 ==
  In1 : Inport
  Compare To Constant1 : simulink/Logic and Bit Operations/Compare To Constant  relop=~=  const=0  OutDataTypeStr=uint8
  Sample & Hold : powerlib_extras/Control  Blocks/Sample & Hold  ic=0
  Out1 : Outport
  Out2 : Outport  Port=2
  wires:
  Sample & Hold/1 -> Out1/1
  In1/1 -> Sample & Hold/1, Compare To Constant1/1
  Compare To Constant1/1 -> Sample & Hold/2, Out2/1

== system autonomous_takeoff_landing/input/Subsystem2/Subsystem4 ==
  In1 : Inport
  Compare To Constant1 : simulink/Logic and Bit Operations/Compare To Constant  relop=~=  const=0  OutDataTypeStr=uint8
  Sample & Hold : powerlib_extras/Control  Blocks/Sample & Hold  ic=0
  Out1 : Outport
  Out2 : Outport  Port=2
  wires:
  Sample & Hold/1 -> Out1/1
  In1/1 -> Sample & Hold/1, Compare To Constant1/1
  Compare To Constant1/1 -> Sample & Hold/2, Out2/1

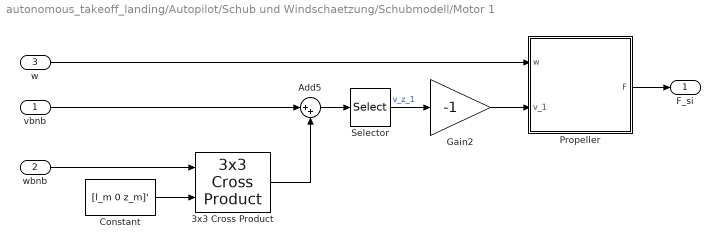
== system autonomous_takeoff_landing/Autopilot/Schub und Windschaetzung/Schubmodell/Motor 1 ==
  vbnb : Inport
  wbnb : Inport  Port=2
  w : Inport  Port=3
  3x3 Cross Product : aerolibutil/3x3 Cross Product
  Add5 : Sum  Inputs=|++
  Constant : Constant  Value=[l_m 0 z_m]'  VectorParams1D=off
  Gain2 : Gain  Gain=-1
  Propeller : Subsystem
  Selector : Selector  InputPortWidth=3  IndexOptions=Index vector (dialog)  Indices=[3]  OutputSizes=1
  F_si : Outport
  wires:
  wbnb/1 -> 3x3 Cross Product/1
  Constant/1 -> 3x3 Cross Product/2
  vbnb/1 -> Add5/1
  3x3 Cross Product/1 -> Add5/2
  Add5/1 -> Selector/1
  Selector/1 -> Gain2/1  "v_z_1"
  Gain2/1 -> Propeller/2(v_1)
  Propeller/1(F) -> F_si/1
  w/1 -> Propeller/1(w)

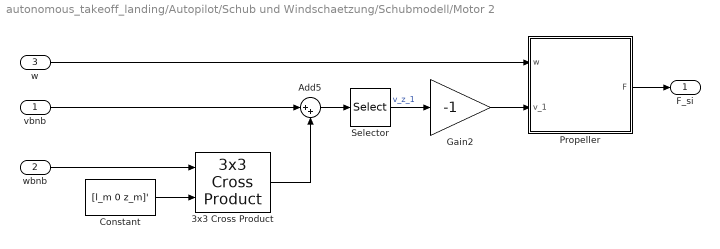
== system autonomous_takeoff_landing/Autopilot/Schub und Windschaetzung/Schubmodell/Motor 2 ==
  vbnb : Inport
  wbnb : Inport  Port=2
  w : Inport  Port=3
  3x3 Cross Product : aerolibutil/3x3 Cross Product
  Add5 : Sum  Inputs=|++
  Constant : Constant  Value=[l_m 0 z_m]'  VectorParams1D=off
  Gain2 : Gain  Gain=-1
  Propeller : Subsystem
  Selector : Selector  InputPortWidth=3  IndexOptions=Index vector (dialog)  Indices=[3]  OutputSizes=1
  F_si : Outport
  wires:
  w/1 -> Propeller/1(w)
  Propeller/1(F) -> F_si/1
  Gain2/1 -> Propeller/2(v_1)
  Selector/1 -> Gain2/1  "v_z_1"
  Add5/1 -> Selector/1
  3x3 Cross Product/1 -> Add5/2
  vbnb/1 -> Add5/1
  Constant/1 -> 3x3 Cross Product/2
  wbnb/1 -> 3x3 Cross Product/1

== system autonomous_takeoff_landing/Autopilot/Schub und Windschaetzung/Schubmodell/Motor 3 ==
  vbnb : Inport
  wbnb : Inport  Port=2
  w : Inport  Port=3
  3x3 Cross Product : aerolibutil/3x3 Cross Product
  Add5 : Sum  Inputs=|++
  Constant : Constant  Value=[l_m 0 z_m]'  VectorParams1D=off
  Gain2 : Gain  Gain=-1
  Propeller : Subsystem
  Selector : Selector  InputPortWidth=3  IndexOptions=Index vector (dialog)  Indices=[3]  OutputSizes=1
  F_si : Outport
  wires:
  wbnb/1 -> 3x3 Cross Product/1
  Constant/1 -> 3x3 Cross Product/2
  vbnb/1 -> Add5/1
  3x3 Cross Product/1 -> Add5/2
  Add5/1 -> Selector/1
  Selector/1 -> Gain2/1  "v_z_1"
  Gain2/1 -> Propeller/2(v_1)
  Propeller/1(F) -> F_si/1
  w/1 -> Propeller/1(w)

== system autonomous_takeoff_landing/Autopilot/Schub und Windschaetzung/Schubmodell/Motor 4 ==
  vbnb : Inport
  wbnb : Inport  Port=2
  w : Inport  Port=3
  3x3 Cross Product : aerolibutil/3x3 Cross Product
  Add5 : Sum  Inputs=|++
  Constant : Constant  Value=[l_m 0 z_m]'  VectorParams1D=off
  Gain2 : Gain  Gain=-1
  Propeller : Subsystem
  Selector : Selector  InputPortWidth=3  IndexOptions=Index vector (dialog)  Indices=[3]  OutputSizes=1
  F_si : Outport
  wires:
  w/1 -> Propeller/1(w)
  Propeller/1(F) -> F_si/1
  Gain2/1 -> Propeller/2(v_1)
  Selector/1 -> Gain2/1  "v_z_1"
  Add5/1 -> Selector/1
  3x3 Cross Product/1 -> Add5/2
  vbnb/1 -> Add5/1
  Constant/1 -> 3x3 Cross Product/2
  wbnb/1 -> 3x3 Cross Product/1

== system autonomous_takeoff_landing/Autopilot/Schub und Windschaetzung/Windabschaetzung/F_g_b ==
  DCMbe : Inport
  F_g_e : Subsystem
  Product1 : Product  Multiplication=Matrix(*)  RndMeth=Zero
  F_g_b : Outport
  wires:
  DCMbe/1 -> Product1/1
  Product1/1 -> F_g_b/1
  F_g_e/1(F_g_e) -> Product1/2

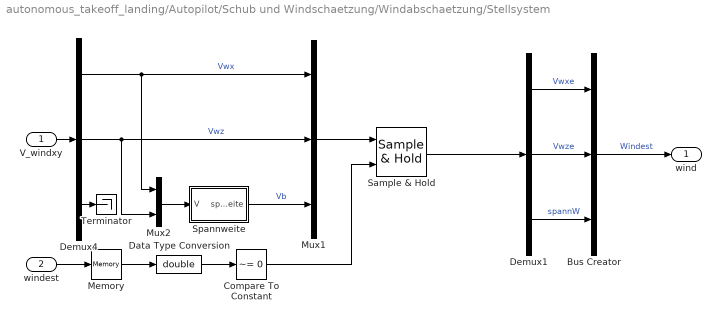
== system autonomous_takeoff_landing/Autopilot/Schub und Windschaetzung/Windabschaetzung/Stellsystem ==
  V_windxy : Inport
  windest : Inport  Port=2
  Bus Creator : BusCreator  Inputs=3
  Compare To Constant : simulink/Logic and Bit Operations/Compare To Constant  relop=~=  const=0  OutDataTypeStr=boolean
  Data Type Conversion : DataTypeConversion  OutDataTypeStr=double  SampleTime=dt
  Demux1 : Demux  Outputs=3
  Demux4 : Demux  Outputs=3
  Memory : Memory
  Mux1 : Mux  Inputs=3
  Mux2 : Mux  Inputs=2
  Sample & Hold : powerlib_extras/Control  Blocks/Sample & Hold  ic=0
  Spannweite : Subsystem
  Terminator : Terminator
  wind : Outport
  wires:
  V_windxy/1 -> Demux4/1
  Mux1/1 -> Sample & Hold/1
  Sample & Hold/1 -> Demux1/1
  Compare To Constant/1 -> Sample & Hold/2
  windest/1 -> Memory/1
  Data Type Conversion/1 -> Compare To Constant/1
  Mux2/1 -> Spannweite/1(V)
  Demux4/2 -> Mux2/2, Mux1/2  "Vwz"
  Demux4/1 -> Mux2/1, Mux1/1  "Vwx"
  Demux4/3 -> Terminator/1
  Spannweite/1(spannweite) -> Mux1/3  "Vb"
  Memory/1 -> Data Type Conversion/1
  Demux1/1 -> Bus Creator/1  "Vwxe"
  Demux1/2 -> Bus Creator/2  "Vwze"
  Demux1/3 -> Bus Creator/3  "spannW"
  Bus Creator/1 -> wind/1  "Windest"

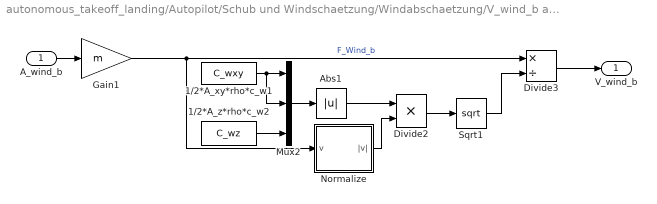
== system autonomous_takeoff_landing/Autopilot/Schub und Windschaetzung/Windabschaetzung/V_wind_b aus A_wind_b ==
  A_wind_b : Inport
  1/2*A_xy*rho*c_w1 : Constant  Value=C_wxy
  1/2*A_z*rho*c_w2 : Constant  Value=C_wz
  Abs1 : Abs
  Divide2 : Product  Inputs=**
  Divide3 : Product  Inputs=*/
  Gain1 : Gain  Gain=m
  Mux2 : Mux  Inputs=3
  Normalize : Subsystem  mask(Quaternion Modulus){}
      mask help: Calculate the modulus of a quaternion.
      mask init:
      | aeroicon('aeroblk');
      mask Help: eval('asbhelp');
  Sqrt1 : Sqrt  SaturateOnIntegerOverflow=on
  V_wind_b : Outport
  wires:
  A_wind_b/1 -> Gain1/1
  Gain1/1 -> Normalize/1(v), Divide3/1  "F_Wind_b"
  Divide3/1 -> V_wind_b/1
  Divide2/1 -> Sqrt1/1
  Sqrt1/1 -> Divide3/2
  1/2*A_xy*rho*c_w1/1 -> Mux2/1, Mux2/2
  1/2*A_z*rho*c_w2/1 -> Mux2/3
  Mux2/1 -> Abs1/1
  Abs1/1 -> Divide2/1
  Normalize/1(|v|) -> Divide2/2

== system autonomous_takeoff_landing/Autopilot/Schub und Windschaetzung/Schubmodell/Motor 1/Propeller ==
  w : Inport
  v_1 : Inport  Port=2
  Divide : Product  Inputs=/*
  Math Function : Math  Operator=square  SaturateOnIntegerOverflow=on
  Polynomial : Polyval  Coefs=[CT3 CT2 CT1 CT0]
  R : Gain  Gain=R
  R1 : Gain  Gain=pi
  R2 : Gain  Gain=rho*pi*R^4
  mult : Product
  F : Outport
  wires:
  R/1 -> Divide/1
  R1/1 -> Divide/2
  Divide/1 -> Polynomial/1  "J"
  Polynomial/1 -> R2/1  "CT"
  R2/1 -> mult/2
  Math Function/1 -> mult/1
  w/1 -> R/1, Math Function/1
  v_1/1 -> R1/1
  mult/1 -> F/1

== system autonomous_takeoff_landing/Autopilot/Schub und Windschaetzung/Schubmodell/Motor 2/Propeller ==
  w : Inport
  v_1 : Inport  Port=2
  Divide : Product  Inputs=/*
  Math Function : Math  Operator=square  SaturateOnIntegerOverflow=on
  Polynomial : Polyval  Coefs=[CT3 CT2 CT1 CT0]
  R : Gain  Gain=R
  R1 : Gain  Gain=pi
  R2 : Gain  Gain=rho*pi*R^4
  mult : Product
  F : Outport
  wires:
  mult/1 -> F/1
  v_1/1 -> R1/1
  w/1 -> Math Function/1, R/1
  Math Function/1 -> mult/1
  R2/1 -> mult/2
  Polynomial/1 -> R2/1  "CT"
  Divide/1 -> Polynomial/1  "J"
  R1/1 -> Divide/2
  R/1 -> Divide/1

== system autonomous_takeoff_landing/Autopilot/Schub und Windschaetzung/Schubmodell/Motor 3/Propeller ==
  w : Inport
  v_1 : Inport  Port=2
  Divide : Product  Inputs=/*
  Math Function : Math  Operator=square  SaturateOnIntegerOverflow=on
  Polynomial : Polyval  Coefs=[CT3 CT2 CT1 CT0]
  R : Gain  Gain=R
  R1 : Gain  Gain=pi
  R2 : Gain  Gain=rho*pi*R^4
  mult : Product
  F : Outport
  wires:
  R/1 -> Divide/1
  R1/1 -> Divide/2
  Divide/1 -> Polynomial/1  "J"
  Polynomial/1 -> R2/1  "CT"
  R2/1 -> mult/2
  Math Function/1 -> mult/1
  w/1 -> R/1, Math Function/1
  v_1/1 -> R1/1
  mult/1 -> F/1

== system autonomous_takeoff_landing/Autopilot/Schub und Windschaetzung/Schubmodell/Motor 4/Propeller ==
  w : Inport
  v_1 : Inport  Port=2
  Divide : Product  Inputs=/*
  Math Function : Math  Operator=square  SaturateOnIntegerOverflow=on
  Polynomial : Polyval  Coefs=[CT3 CT2 CT1 CT0]
  R : Gain  Gain=R
  R1 : Gain  Gain=pi
  R2 : Gain  Gain=rho*pi*R^4
  mult : Product
  F : Outport
  wires:
  mult/1 -> F/1
  v_1/1 -> R1/1
  w/1 -> Math Function/1, R/1
  Math Function/1 -> mult/1
  R2/1 -> mult/2
  Polynomial/1 -> R2/1  "CT"
  Divide/1 -> Polynomial/1  "J"
  R1/1 -> Divide/2
  R/1 -> Divide/1

== system autonomous_takeoff_landing/Autopilot/Schub und Windschaetzung/Windabschaetzung/F_g_b/F_g_e ==
  Mux : Mux  Inputs=3
  mg_x : Constant  Value=0
  mg_y : Constant  Value=0
  mg_z : Constant  Value=m*g
  F_g_e : Outport
  wires:
  mg_x/1 -> Mux/1
  mg_y/1 -> Mux/2
  mg_z/1 -> Mux/3
  Mux/1 -> F_g_e/1

== system autonomous_takeoff_landing/Autopilot/Schub und Windschaetzung/Windabschaetzung/Stellsystem/Spannweite ==
  V : Inport
  Constant : Constant  Value=0
  Terminator : Terminator
  spannweite : Outport
  wires:
  V/1 -> Terminator/1
  Constant/1 -> spannweite/1

== system autonomous_takeoff_landing/Autopilot/Schub und Windschaetzung/Windabschaetzung/V_wind_b aus A_wind_b/Normalize ==
  v : Inport
  Norm : Subsystem  mask(Quaternion Norm){}
      mask help: Calculate the norm of a quaternion.
      mask init:
      | aeroicon('aeroblk');
      mask Help: eval('asbhelp');
  sqrt : Sqrt  AlgorithmType=Newton-Raphson  SaturateOnIntegerOverflow=on
  |v| : Outport
  wires:
  Norm/1(norm(v)) -> sqrt/1
  v/1 -> Norm/1(v)
  sqrt/1 -> |v|/1

== system autonomous_takeoff_landing/Autopilot/Schub und Windschaetzung/Windabschaetzung/V_wind_b aus A_wind_b/Normalize/Norm ==
  v : Inport
  Product3 : Product  Multiplication=Matrix(*)
  Reshape : Reshape  OutputDimensionality=Row vector (2-D)
  Reshape1 : Reshape  OutputDimensionality=Column vector (2-D)
  norm(v) : Outport
  wires:
  Reshape/1 -> Product3/1
  Reshape1/1 -> Product3/2
  Product3/1 -> norm(v)/1
  v/1 -> Reshape1/1, Reshape/1

== matlab function Autopilot/MATLAB Function1 ==
  data: u input double; y output double
function y = fcn(u)
persistent i;
if isempty(i)
    i=0;
end
persistent ualt;
if isempty(ualt)
    ualt=0;
end


if i== 50
    i=0;
    y=u;
else
    i=i+1;
    y=ualt;
end

end

== matlab function Autopilot/MATLAB Function ==
  data: u input double; y output double
function y = fcn(u)
persistent i;
if isempty(i)
    i=0;
end
persistent ualt;
if isempty(ualt)
    ualt=0;
end


if i== 50
    i=0;
    y=u;
else
    i=i+1;
    y=ualt;
end

end

== matlab function Autopilot/MATLAB Function2 ==
  data: u input double; y output double
function y = fcn(u)
persistent i;
if isempty(i)
    i=0;
end
persistent ualt;
if isempty(ualt)
    ualt=0;
end


if i== 50
    i=0;
    y=u;
else
    i=i+1;
    y=ualt;
end

end

== stateflow chart Autopilot/Zustandsautomat1 ==
  settings: sampleTime=0.01  executeAtInitialization=1
  state position_hold/
    en:	reglerwahl=1;
    sollwert[2]=hFlug,
    auto=0;
    ex: 	sollwert=0;
    sollwert[0]=messwert[0];
    sollwert[1]=messwert[1];
    sollwert[2]=hFlug;
  state amBoden/
    state Selbstcheck/
      en:	reglerwahl[5] = 1;
    state error/
      en: 	reglerwahl=0;
      auto=0;
      windest=0;
      Schub=0;
      diagnose[3]=1;
      ex:	diagnose=0;
      error -> error [order 1] : [state[5]<Bstart]
          | /diagnose[1]=1
    state Standby/
      en:	windest=0;
      auto=0;
      reglerwahl=0;
      boden[0]=messwert[0];
      boden[1]=messwert[1];
      boden[2]=messwert[3];
      boden[3]=messwert[4];
    error -> Standby [order 1] : [hasChanged(state[0])&&state[0]==1]
        | {auto[0]=1;}/debug=0;
    Selbstcheck -> error : after(60,sec)
        | /diagnose[2]=1;
    Standby -> Selbstcheck : [state[0]==1&&state[2]==1]
        | {auto[0]=1;i=0}
    (default) -> Standby : /Schub=0;
  state landen/
    state pos_anfliegen
    state sinkflug/
      en: 	windest=1;
      reglerwahl[3]=1;
    state landen
    state windcheck/
    landen.landen -> sinkflug [order 3] : [!lagetol(messwert)&&state[5]>Bkrit]
        | {sollwert[2]=hLanden+dhSinkflug;}
    (default) -> pos_anfliegen
    sinkflug -> landen.landen [order 2] : [messwert[12]<hLanden]
        | {reglerwahl[3]=0;;windest=0;}
    pos_anfliegen -> windcheck : [postol(sollwert,messwert)]
    landen.landen -> landen.landen [order 2] : [abs(messwert[12]-sollwert[2])<dhZulSinkflug&&abs(messwert[8])<zpLanden/2]
        | {sollwert[2]=sollwert[2]-dhSinkflug;}
    sinkflug -> sinkflug [order 3] : [abs(messwert[12]-sollwert[2])<dhZulSinkflug&&abs(messwert[8])<zpLanden]
        | {sollwert[2]=sollwert[2]-dhSinkflug;}
    windcheck -> pos_anfliegen [order 1] : [!postol(sollwert,messwert)]
    windcheck -> (junction 44) [order 2] : after(twc,sec)
    (junction 44) -> sinkflug [order 1] : [wind(messwert)&&lagetol(messwert)]
    (junction 44) -> windcheck [order 2] : /diagnose[0]=1;
    sinkflug -> pos_anfliegen [order 1] : [!postol(sollwert,messwert)||!lagetol(messwert)||!wind(messwert)]
  state starten/
    state hochfahren/
    state abheben/
      en:	sollwert[2]	=hFlug;
      reglerwahl[1]=1;
      reglerwahl[2]=1;
    (default) -> hochfahren : /reglerwahl[0]=1;
    hochfahren -> hochfahren [order 5] : after(dtStart,sec)
        | [Schub<SchubStart&&abs(messwert[8])<zpStart]{debug[7]=1;}
        | /Schub=Schub+dSchubStart;
    hochfahren -> abheben [order 4] : [state[4]==1]
    hochfahren -> (junction 43) [order 1] : after(dtStart*20,sec){debug[6]=1;}
    abheben -> (junction 43) [order 2] : [!lagetol(messwert)]
    hochfahren -> (junction 43) [order 3] : [!lagetol(messwert)]
        | {debug[4]=1;}
    hochfahren -> (junction 43) [order 2] : [state[0]==0]{debug[5]=1;}
  position_hold -> (junction 45) [order 3] : [state[1]==1&&state[2]==1]
  (default) -> (junction 42)
  abheben -> position_hold [order 1] : [messwert[18]>=hFlug]
      | {windest=1;}
  error -> starten [order 2] : after(tAnlauf,sec)[motor(messwert)&&state[3]==1]
      | {diagnose[2]=0;}
  position_hold -> abheben [order 2] : [messwert[18]<hFlug/2]
  (junction 43) -> error : /
  landen.landen -> amBoden [order 1] : [sollwert[2]<LGH*2&&messwert[12]<LGH*2]
      | {sollwert[2]=0;reglerwahl=0;reglerwahl[0]=1;}
  (junction 42) -> position_hold [order 2] : [state[4]==1]
  landen -> position_hold : [state[1]==0]/diagnose[4]=1;
  position_hold -> (junction 45) [order 1] : [state[5]<Bkrit]
      | {diagnose[5]=1;}
  (junction 42) -> amBoden [order 1] : [state[4]==0]
  (junction 45) -> landen : /diagnose[4]=0;auto[1]=1;
  data: par function_input double size=1; par_angepasst function_output double; n function_input double; b function_output boolean size=1; zul_dmotor parameter double; messwert function_input double size=20; data temporary double; b function_output boolean; messwert function_input double size=20; zul_win parameter double; messwert function_input double size=20; b function_output boolean; zul_dwmax parameter double; zul_w parameter double; sollwert function_input double size=9; b function_output boolean; messwert function_input double size=20; zul_dp parameter double; Schub output double size=1 =0; messwert input double; state input double; i local double size=1 =0; sollwert output double size=9 =[X_start Y_start Z_start 0 0 0 0 0 0 ]; reglerwahl output double size=6 =[0 0 0 0 0 0]; auto output double size=3 =[0 0 0]; Standby output boolean; Selbstcheck output boolean; hochfahren output boolean; abheben output boolean; dSchubLanden parameter double; SchubStart parameter double; dhSinkflug parameter double; dhZulSinkflug parameter double; hFlug parameter double; hLanden parameter double; dtStart parameter double; twc parameter double; zpLanden parameter double; dSchubStart parameter double; LGH parameter double; Bstart parameter double; Bkrit parameter double; tAnlauf parameter double; SchubRun parameter double; Bsafe parameter double; boden local double size=4 =[0 0 0 0]; zpStart parameter double; position_hold output boolean; pos_anfliegen output boolean; windcheck output boolean; sinkflug output boolean; landen output boolean; error output boolean; debug output double size=10 =0; diagnose output double size=6 =[0 0 0 0 0 0]; windest output double
  data i settings: description=zählvariable
  events: takt input EITHER_EDGE_EVENT; step local EITHER_EDGE_EVENT
  function par_angepasst=ladestand(par,n):
    | function par_angepasst=ladestand(par,n)
    | 
    | faktor=(Bsafe-state(6))/(Bsafe-Bkrit);
    | 
    | if      state(6)>=Bsafe;
    |     par_angepasst=par;
    | elseif  state(6)<Bkrit && n>0;
    |     par_angepasst=n*par;
    | elseif  state(6)<Bkrit && n==0;
    |     par_angepasst=inf;
    | else    state(6)<Bsafe;
    |     par_angepasst=par+par*faktor^2;
    | end
    | 
    | end
  function b=motor(messwert):
    | function b=motor(messwert)
    | 
    | ist=messwert(16:17);
    | schnell=max(ist);
    | lahm=min(ist);
    | spannweite=schnell-lahm;
    | 
    | if spannweite < 20
    |     b=true;
    | else
    |     b=false;
    | end
    | end
  function b=lagetol(messwert):
    | function b=lagetol(messwert)
    | 
    | % 
    | % zul_win=ladestand(zul_win,2);
    | 
    | pitch=abs(messwert(4));
    | roll=abs(messwert(5));
    | 
    | if (pitch>zul_win)||(roll>zul_win) 
    |     b=false;
    |     debug(1)=pitch;
    |     debug(2)=roll;
    |     
    | else
    |     b=true;
    |     debug(1)=zul_win;
    |     debug(2)=1;
    | end
    | end
  function b=wind(messwert):
    | function b=wind(messwert)
    | 
    | dw=messwert(20);
    | w=sqrt(messwert(18)^2+messwert(19)^2);
    | 
    | zul_dwmax_angepasst=ladestand(zul_dwmax,0);
    | zul_w_angepasst=ladestand(zul_w,0);
    | 
    | if dw < zul_dwmax_angepasst||w<zul_w
    | 	b=true;
    | else
    |     b=false;
    | end
    | end
  function b=postol(sollwert,messwert):
    | function b=postol(sollwert,messwert)
    | 
    | zul_dp_angepasst=ladestand(zul_dp,2);
    | 
    | if (abs(sollwert(1)-messwert(1))<zul_dp_angepasst)&&(abs(sollwert(2)-messwert(2))<zul_dp_angepasst) 
    |     b=true;
    | else
    |     b=false;
    | end
    | end
